simulink model "lsys5"  (R2020b)
settings: Solver=VariableStepAuto  StartTime=0.0  StopTime=10.0  RelTol=1e-3
settings Model: Creator=반달  LastModifiedBy=반달
settings DataIOCC: ReturnWorkspaceOutputs=off

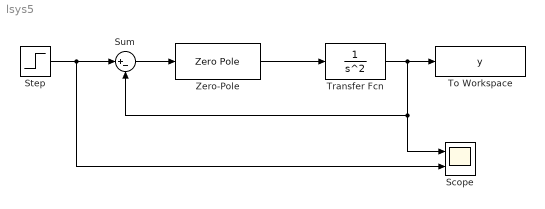
== system lsys5 ==
  Scope : Scope  NumInputPorts=2
  Step : Step  Time=3  SampleTime=0
  Sum : Sum  Inputs=|+-
  To Workspace : ToWorkspace  VariableName=y  SaveFormat=Structure With Time  SampleTime=-1
  Transfer Fcn : TransferFcn  Denominator=[1 0 0]
  Zero-Pole : ZeroPole  Zeros=[-1]  Poles=[-3]  Gain=8
  wires:
  Step/1 -> Scope/2, Sum/1
  Sum/1 -> Zero-Pole/1
  Zero-Pole/1 -> Transfer Fcn/1
  Transfer Fcn/1 -> Scope/1, Sum/2, To Workspace/1
